simulink model "controller_stateflow_2021a"  (R2021a)
settings: Solver=FixedStepAuto  StartTime=0.0  StopTime=inf  FixedStep=0.05  RelTol=1e-3
PreLoadFcn:
  | rosinit();
model workspace (MAT data in the model file):
  SL_ROS_VariableLengthArrays_MaxSizes : object (value not decoded)
  pitch = -10
  restart = 0
values from neighbouring files (symbols this model uses):
  Pose = distance*inv(toPandatf)*Pose_d0    [inverseContoller3.m]    (also in inverseContoller4.m = distance*inv(toUR10etf)*Point_d0; inverseContoller_dual.m = inv(toUR10etf)*Point_d0; inverseContoller_dual2.m = inv(toUR10etf)*Point_d0)
undefined symbols (not defined in the file or in its folder): StartTime
libraries: robotlib x19, robotmaniplib x5, robotcorelib x3, robotgazebolib x1
(part 2 of 2)

== matlab function controller_stateflow_2021a/MATLAB Function14 ==
  data: enable output; msgOut output Bus: SL_Bus_controller_stateflow_SetModelStateRequest_4q9jrn; msgIn input Bus: SL_Bus_controller_stateflow_SetModelStateRequest_4q9jrn; state input; boxPose input Bus: SL_Bus_controller_stateflow_geometry_msgs_Pose
function [enable,msgOut]  = fcn(msgIn,state,boxPose)

    msgOut = msgIn;
    
    bodyname = 'box_38_18_14';
    enable = 1;
    
    
    lenName = uint32(length(bodyname));
    msgOut.ModelState.ModelName(1:lenName,1) = uint8(convertStringsToChars(bodyname))';
    msgOut.ModelState.ModelName_SL_Info.CurrentLength = uint32(lenName);
   
    msgOut.ModelState.Pose = boxPose;

%     msgOut.ModelState.Twist.Linear.X=1.;
    
    msgOut.ModelState.Pose.Position.X = msgOut.ModelState.Pose.Position.X +0.02;


end
 

 
 
% enable = 0;
% y=0;
% 
% bodyname = 'box_38_18_14::link_0';
% lenName = uint32(length(bodyname));
% msgOut.BodyName_SL_Info.CurrentLength = uint32(lenName);
% msgOut.BodyName(1:lenName,1) = uint8(convertStringsToChars(bodyname))';
% 
% refname = 'iliad::ur10e_wrist_3_link';
% lenName = uint32(length(refname));
% msgOut.ReferenceFrame(1:lenName,1) = uint8(convertStringsToChars(refname))';
% msgOut.ReferenceFrame_SL_Info.CurrentLength = uint32(lenName);
% 
% msgOut.Wrench.Force.Y = 0;
% 
% if state == 12 && coll == 1
%     msgOut.Wrench.Force.Y = 0;
% 
%     msgOut.Wrench.Force.Z = -380;
% 
%     y=-0.0;
% end

== matlab function controller_stateflow_2021a/MATLAB Function2 ==
  data: u input; y output double
function y = fcn(u)
y=0;
if u.Sec >= 1
y=1;
end

== matlab function controller_stateflow_2021a/Chart3/get_panda_pose_track/MATLAB Function ==
  data: Pose output; boxPos input; boxZYX input; sumPos input; sumZYX input; panda_state input; Weights output; initialGuess output; state input
function [Pose, Weights, initialGuess] = fcn(boxPos,boxZYX,sumPos,sumZYX,panda_state,state)

dimBox_x=0.38;
dimBox_y=0.18;
dimBox_z=0.14;

toSumChapa = [0;0;0.51];
toFranka = [0.25;-0.22;0.15];

boxPos_offset = [0;0;0];

boxtf_01 = [[eul2rotm(boxZYX', 'ZYX')],boxPos; ...
            0 0 0                               1           ];


if state == 122
    boxPos_offset = [0;+dimBox_y/2-0.05;dimBox_z/2+0.035];
end



% boxPos0 = boxPos+boxPos_offset;

boxPos0 = boxtf_01*[boxPos_offset;1];

sumtf_01 = [[eul2rotm(sumZYX', 'ZYX')],sumPos; ...
            0 0 0                               1           ];
sumtopandatf_12 = [[eul2rotm([0,pi/4,0], 'ZYX')],toSumChapa+toFranka; ...
            0 0 0                               1           ];

toPandatf = sumtf_01*sumtopandatf_12;

boxx = inv(toPandatf)*[boxPos0(1:3);1];


Pose = [[eul2rotm([pi,0,0], 'ZYX')],[boxx(1);boxx(2);boxx(3)]; ...
            0 0 0                               1           ];
if state == 122
    Pose = [[eul2rotm([pi,pi/8,0], 'ZYX')],[boxx(1);boxx(2);boxx(3)]; ...
            0 0 0                               1           ];
end

Weights = [1,1,1,1,1,1];


initialGuess = panda_state;

end

== matlab function controller_stateflow_2021a/MATLAB Function12 ==
  data: enable output; msgOut output Bus: SL_Bus_controller_stateflow_ApplyBodyWrenchRequest_gxwnto; msgIn input Bus: SL_Bus_controller_stateflow_ApplyBodyWrenchRequest_gxwnto; state input; coll input; T_ur_velvCnt input
function [enable,msgOut]  = fcn(msgIn,state,coll,T_ur_velvCnt)

    msgOut = msgIn;
    
    bodyname = 'box_38_18_14::link_0';
    enable = 0;
    
    lenName = uint32(length(bodyname));
    msgOut.BodyName(1:lenName,1) = uint8(convertStringsToChars(bodyname))';
    msgOut.BodyName_SL_Info.CurrentLength = uint32(lenName);
   
    msgOut.ReferenceFrame(1:lenName,1) = uint8(convertStringsToChars(bodyname))';
    msgOut.ReferenceFrame_SL_Info.CurrentLength = uint32(lenName);
    
    msgOut.Wrench.Force.X =  0;
    msgOut.Wrench.Force.Y =  0;
    msgOut.Wrench.Force.Z =  0;
    msgOut.Wrench.Torque.X = 0;
    msgOut.Wrench.Torque.Y = 0;
    msgOut.Wrench.Torque.Z = 0;
        
    F_v = [0;0;0;1];

    if state == 1 && coll == 1
        k=0.3;
        F_v = [0;0;-80*k;1];

        msgOut.Wrench.Torque.X = 0;
        msgOut.Wrench.Torque.Y = 0;
        msgOut.Wrench.Torque.Z = 0;

        msgOut.ReferencePoint.X = 0;
        msgOut.ReferencePoint.Y = 0;
        msgOut.ReferencePoint.Z = 0;
        
        msgOut.Duration.Sec = 0;
        msgOut.Duration.Nsec = 1e7;

        fprintf("lo tirooo \n");

        enable = 1;
    end


    if state == -1
        k=0.8;
        F_v = [0;0;80*k;1];

        msgOut.Wrench.Torque.X = 0;
        msgOut.Wrench.Torque.Y = 0;
        msgOut.Wrench.Torque.Z = 0;
        
        msgOut.ReferencePoint.X = 0;
        msgOut.ReferencePoint.Y = 0;
        msgOut.ReferencePoint.Z = 0;

        msgOut.Duration.Sec = 0;
        msgOut.Duration.Nsec = 1e7;

        fprintf("lo lancioo \n");

        enable = 1;        
    end
        
    F_w = T_ur_velvCnt*F_v;

    msgOut.Wrench.Force.X = F_w(1);
    msgOut.Wrench.Force.Y = F_w(2);
    msgOut.Wrench.Force.Z = F_w(3);

end

== matlab function controller_stateflow_2021a/Subsystem/MATLAB Function1 ==
  data: Time input; msgOut output Bus: SL_Bus_controller_stateflow_trajectory_msgs_JointTrajectory; msgIn input; msgPoint input; Points input; TimeFromStart input
function msgOut   = fcn(Time, msgIn, msgPoint, Points,TimeFromStart)

    msgOut = msgIn;
    if Time.Sec ~= 0

        jointNames = {'ur10e_shoulder_pan_joint','ur10e_shoulder_lift_joint','ur10e_elbow_joint'...
            'ur10e_wrist_1_joint','ur10e_wrist_2_joint','ur10e_wrist_3_joint'};
        numJoints = uint32(length(jointNames));
        msgOut.JointNames_SL_Info.CurrentLength = numJoints;
        for idx = 1:numJoints
            jName = jointNames{idx};
            lenName = uint32(length(jName));
            msgOut.JointNames(idx).Data(1:lenName) = uint8(jName);
            msgOut.JointNames(idx).Data_SL_Info.CurrentLength = lenName;
        end
        
        msgOut.Points = msgPoint;
        msgOut.Points.Positions(1:6) = Points(1:6,1);
        msgOut.Points.Positions_SL_Info.CurrentLength = uint32(6);

        msgOut.Points.Velocities(1:6) = [0 ;0 ;0 ;0 ;0 ;0];
        msgOut.Points.Velocities_SL_Info.CurrentLength = uint32(6);
        
        msgOut.Points.Accelerations(1:6) = [0 ;0 ;0 ;0 ;0 ;0];
        msgOut.Points.Accelerations_SL_Info.CurrentLength = uint32(6);
        
        msgOut.Points.Effort(1:6) = [0 ;0 ;0 ;0 ;0 ;0];
        msgOut.Points.Effort_SL_Info.CurrentLength = uint32(6);

        msgOut.Header.Stamp.Sec = Time.Sec;
        msgOut.Header.Stamp.Nsec = Time.Nsec;
        
        msgOut.Header.Seq = uint32(0);

        msgOut.Points.TimeFromStart.Sec = TimeFromStart;
        msgOut.Points.TimeFromStart.Nsec = 0;
        msgOut.Points_SL_Info.CurrentLength = uint32(1);
    end
end

== matlab function controller_stateflow_2021a/Subsystem5/MATLAB Function4 ==
  data: x output; T input; y output; box input; z output; sumPos input; sumZYX input; T_ur_velvCnt output; coll output; boxx output
function [x,y,z,T_ur_velvCnt,coll,boxx] = fcn(T,box,sumPos,sumZYX)
    
    dimBox = [0.38;0.18;0.14];
    
    toSumChapa = [0;0;0.51];
    toUR10e = [0.35;0.32;0.05];
    
    velvet_length = 0.28+0.04;
    velvet_height = 0.08;
    
    base_ur_offset = [0;0;0.05];
    
    sumtf_01 = [[eul2rotm(sumZYX', 'ZYX')],sumPos; ...
                0 0 0                               1           ];
    sumtoUR10etf_12 = [[eul2rotm([0,0,0], 'ZYX')],toSumChapa+toUR10e+base_ur_offset; ...
                0 0 0                               1           ];
    
    toUR10etf = sumtf_01*sumtoUR10etf_12;
    
    to_velvCnt = [[eul2rotm([0,0,0], 'ZYX')],[0;-velvet_height/2-dimBox(3)/2;velvet_length-dimBox(2)/2]; ...
                0 0 0                               1           ];
    
    T_ur_velvCnt = toUR10etf*T*to_velvCnt;
    
    boxx = inv(T_ur_velvCnt)*[box;1];
    
    x = boxx(1);
    y = boxx(2);
    z = boxx(3);
    
    coll = 0;
    
    goal = [0;0;0.165];
    tol = [0.05;0.05;0.0];
    
    if boxx(1) <= goal(1) + tol(1) && boxx(1) >= goal(1) - tol(1) && ...
       boxx(2) <= goal(2) + tol(2) && boxx(2) >= goal(2) - tol(2) && ...
       boxx(3) <= goal(3) - tol(3)
            coll = 1;
    end



end

== matlab function controller_stateflow_2021a/Subsystem5/MATLAB Function6 ==
  data: u input; y output
function y = fcn(u)

y = u(1:6);

== matlab function controller_stateflow_2021a/Subsystem5/MATLAB Function7 ==
  data: box_ok output; x input; y input; z input; tol input; box_off output
function [box_ok,box_off]  = fcn(x,y,z,tol)


    dimBox_x=0.38;
    dimBox_y=0.18;
    dimBox_z=0.14;
    velvet_length = 0.28+0.04;
    goal =[0,0,0];

    box_ok = 0;

    box_off = 0;

    if  z <= 0

        box_ok=1;

    end

    if  z >= 0.17

        box_off=1;

    end


end
